simulink model "RM3_Hydraulic_PTO_HeavingSurging4"  (R2019b)
settings: Solver=ode14x  StartTime=0  StopTime=250  FixedStep=0.01  MaxStep=0.01  RelTol=1e-3  EnableMultiTasking=on
values from neighbouring files (symbols this model uses):
  simu = simulationClass()    [wecSimInputFile.m]
  waves = waveClass('regular')    [wecSimInputFile.m]
undefined symbols (not defined in the file or in its folder): body, constraint, pto, X, Y, Z
libraries: nesl_utility x73, sm_lib x40, WECSim_Lib x8, vrlib x1
(part 4 of 4)

== matlab function RM3_Hydraulic_PTO_HeavingSurging4/buoy/Hydrodynamic Body/Nonlinear Wave Elevation/Linear or Instantaneous Free Surface/Instantaneous Water Free Surface  /Instantaneous FS ==
  data: x input; center input; f output; cg input; AH input; w input; dw input; k input; typeNum input; t input; rampT input; phaseRand input; waveDir input
function f  = waveElevation(x,center,cg,AH,w,dw,k,typeNum,t,rampT,phaseRand,waveDir)
% Function to calculate the wave elevation at the ceontroids of triangulated surface
% NOTE: This function assumes that the STL file is imported with its CG at 0,0,0
f = calc_elev(x,center,cg,AH,w,dw,k,typeNum,t,rampT,phaseRand, waveDir);
end

function f = calc_elev(x,center,cg,AH,w,dw,k,typeNum,t,rampT,phaseRand,waveDir)
% Function to rotate and translate body and call wave elevation function at new locations

% Compute new tri center coords after cog rotation and translation
center = rotateXYZ(center,[1 0 0],x(4));
center = rotateXYZ(center,[0 1 0],x(5));
center = rotateXYZ(center,[0 0 1],x(6));
center = offsetXYZ(center,x);
center = offsetXYZ(center,cg);
% Calculate the free surface
f=waveElev(center,AH,w,dw,t,k,rampT,phaseRand,typeNum,waveDir);
end

function verts = offsetXYZ(verts,x)
% Function to move the position vertices
verts(:,1) = verts(:,1) + x(1);
verts(:,2) = verts(:,2) + x(2);
verts(:,3) = verts(:,3) + x(3);
end

function xn = rotateXYZ(x,ax,t)
% Function to rotate a point about an arbitrary axis
% x: 3-component coordinates
% ax: axis about which to rotate (must be a vector length 1)
% t: rotation angle
% xn: new coordinates after rotation
rotMat = zeros(3);
rotMat(1,1) = ax(1)*ax(1)*(1-cos(t))    + cos(t);
rotMat(1,2) = ax(2)*ax(1)*(1-cos(t))    + ax(3)*sin(t);
rotMat(1,3) = ax(3)*ax(1)*(1-cos(t))    - ax(2)*sin(t);
rotMat(2,1) = ax(1)*ax(2)*(1-cos(t))    - ax(3)*sin(t);
rotMat(2,2) = ax(2)*ax(2)*(1-cos(t))    + cos(t);
rotMat(2,3) = ax(3)*ax(2)*(1-cos(t))    + ax(1)*sin(t);
rotMat(3,1) = ax(1)*ax(3)*(1-cos(t))    + ax(2)*sin(t);
rotMat(3,2) = ax(2)*ax(3)*(1-cos(t))    - ax(1)*sin(t);
rotMat(3,3) = ax(3)*ax(3)*(1-cos(t))    + cos(t);
xn = x*rotMat;
end

function f=waveElev(center,AH,w,dw,t,k,rampT,phaseRand,typeNum,waveDir)
% Function to calculate the wave elevation at an array of points
f = zeros(length(center(:,3)),1);
cx = center(:,1);
cy = center(:,2);
X = cx*cos(waveDir*pi/180) + cy*sin(waveDir*pi/180);
if typeNum <10
elseif typeNum <20
    f = AH(1).*cos(k(1).*X-w(1)*t);
elseif typeNum <30
    tmp=sqrt(AH.*dw);
    tmp1 = ones(1,length(center(:,1)));
    tmp2 = (w.*t+phaseRand)*tmp1;
    tmp3 = cos(k*X'- tmp2);
    f(:,1) = tmp3'*tmp;
end
if t<=rampT
    rampF = (1+cos(pi+pi*t/rampT))/2;
    f = f.*rampF;
end
end

== matlab function RM3_Hydraulic_PTO_HeavingSurging4/buoy/Hydrodynamic Body/Structure/Motion Sensor/Angle ==
  data: Q input; E output
function E  = quaternion2eulerxyz(Q)
% Takes the orientation of the body in quaternion format and converts it to
% Euler/Tait-Bryan/Cardan angles in the XYZ convention: roll [-180,180],
% followed by pitch [-90,90], followed by yaw [-180,180].
E = zeros(3,1);

E(1) = atan2(-2 * ( Q(3)*Q(4) - Q(1)*Q(2)), (Q(1)^2 - Q(2)^2 - Q(3)^2 + Q(4)^2));
E(2) = asin(2 *   ( Q(2)*Q(4) + Q(1)*Q(3)));
E(3) = atan2(-2 * ( Q(2)*Q(3) - Q(1)*Q(4)), (Q(1)^2 + Q(2)^2 - Q(3)^2 - Q(4)^2));

% E(1) = atan2((2*(Q(1)*Q(2)+Q(3)*Q(4))),(1-2*(Q(2)^2+Q(3)^2)));
% E(2) = asin(2*(Q(1)*Q(3)-Q(4)*Q(2)));
% E(3) = atan2((2*(Q(1)*Q(4)+Q(2)*Q(3))),(1-2*(Q(3)^2+Q(4)^2)));

== matlab function RM3_Hydraulic_PTO_HeavingSurging4/buoy/Hydrodynamic Body/Wave Diffraction and Excitation Force Calculation/Linear Wave Excitation Force Variant Subsystem/Irregular Wave Excitation Force/MATLAB Function ==
  data: A input; Fext output; w input; fExtRE input; fExtIM input; phaseRand input; dw input; time input; WaveDir input; WaveSpread input; fExtMD input
function Fext = fcn(A,w,fExtRE,fExtIM,phaseRand,dw,time,WaveDir,WaveSpread,fExtMD)
%#codegen

% pversistent A1 B1 B11 C1 D1 D11 E1 E11

A1=bsxfun(@plus,w*time,pi/2);
Fext = zeros(1,6);
for ii=1:length(WaveDir)
    B1= sin(bsxfun(@plus,A1,phaseRand(:,ii)));
    B11 = sin(bsxfun(@plus,w*time,phaseRand(:,ii)));
    C0 = bsxfun(@times,A*WaveSpread(ii),dw);
    C1 = sqrt(bsxfun(@times,A*WaveSpread(ii),dw));
    D0 =bsxfun(@times,squeeze(fExtMD(ii,:,:)),C0);
    D1 =bsxfun(@times,squeeze(fExtRE(ii,:,:)),C1);
    D11 = bsxfun(@times,squeeze(fExtIM(ii,:,:)),C1);
    E1 = D0+ bsxfun(@times,B1,D1);
    E11 = bsxfun(@times,B11,D11);
    Fext = Fext + sum(bsxfun(@minus,E1,E11));
end

== matlab function RM3_Hydraulic_PTO_HeavingSurging4/buoy/Hydrodynamic Body/Wave Diffraction and Excitation Force Calculation/Nonlinear FK Force Variant Subsystem/With Nonlinear FroudeKrylov Force/Diffraction and Excitation Forces ==
  data: x input; elv input; center input; f output; tnorm input; area input; rho input; g input; cg input; AH input; w input; dw input; wDepth input; deepWaterWave input; k input; typeNum input; t input; phaseRand input; wp output; wpMeanFS output
function [f, wp, wpMeanFS]  = nonFKForce(x,elv,center,tnorm,area,rho,g,cg,AH,w,dw,wDepth,deepWaterWave,k,typeNum,t,phaseRand)
% Function to calculate wave exitation force and moment on a triangulated surface
% NOTE: This function assumes that the STL file is imported with its CG at 0,0,0

% Logic to calculate nonFKForce at reduced sample time
[f, wp, wpMeanFS] = calc_force(x,elv,center,tnorm,area,rho,g,cg,AH,w,dw,wDepth,deepWaterWave,k,typeNum,t,phaseRand);
end

function [f, wp, wpMeanFS]  = calc_force(x,elv,center,tnorm,area,rho,g,cg,AH,w,dw,wDepth,deepWaterWave,k,typeNum,t,phaseRand)
% Function to apply translation and rotation, and calculate forces.

% Compute new tri coords after cog rotation and translation
centerMeanFS = offsetXYZ(center,cg);
avMeanFS     = tnorm .* [area area area];

% Compute new tri coords after cog rotation and translation
center = rotateXYZ(center,[1 0 0],x(4));
center = rotateXYZ(center,[0 1 0],x(5));
center = rotateXYZ(center,[0 0 1],x(6));
center = offsetXYZ(center,x);
center = offsetXYZ(center,cg);
% Compute new normal vectors coords after cog rotation and translation
tnorm = rotateXYZ(tnorm,[1 0 0],x(4));
tnorm = rotateXYZ(tnorm,[0 1 0],x(5));
tnorm = rotateXYZ(tnorm,[0 0 1],x(6));

% Copute area vectors
av = tnorm .* [area area area];

% Calculate the free surface
wpMeanFS=pDis(centerMeanFS,       0,AH,w,dw,wDepth,deepWaterWave,t,k,phaseRand,typeNum,rho,g);
wp      =pDis(center      ,     elv,AH,w,dw,wDepth,deepWaterWave,t,k,phaseRand,typeNum,rho,g);

% Calculate forces
f_linear   =FK(centerMeanFS,       cg,avMeanFS,wpMeanFS);
f_nonLinear=FK(center      ,x(1:3)+cg,av      ,wp      );
f = f_nonLinear-f_linear;
end

function verts = offsetXYZ(verts,x)
% Function to move the position vertices
verts(:,1) = verts(:,1) + x(1);
verts(:,2) = verts(:,2) + x(2);
verts(:,3) = verts(:,3) + x(3);
end

function xn = rotateXYZ(x,ax,t)
% Function to rotate a point about an arbitrary axis
% x: 3-componenet coordinates
% ax: axis about which to rotate (must be a vector length 1)
% t: rotation angle
% xn: new coordinates after rotation
rotMat = zeros(3);
rotMat(1,1) = ax(1)*ax(1)*(1-cos(t))    + cos(t);
rotMat(1,2) = ax(2)*ax(1)*(1-cos(t))    + ax(3)*sin(t);
rotMat(1,3) = ax(3)*ax(1)*(1-cos(t))    - ax(2)*sin(t);
rotMat(2,1) = ax(1)*ax(2)*(1-cos(t))    - ax(3)*sin(t);
rotMat(2,2) = ax(2)*ax(2)*(1-cos(t))    + cos(t);
rotMat(2,3) = ax(3)*ax(2)*(1-cos(t))    + ax(1)*sin(t);
rotMat(3,1) = ax(1)*ax(3)*(1-cos(t))    + ax(2)*sin(t);
rotMat(3,2) = ax(2)*ax(3)*(1-cos(t))    - ax(1)*sin(t);
rotMat(3,3) = ax(3)*ax(3)*(1-cos(t))    + cos(t);
xn = x*rotMat;
end

function f=pDis(center,elv,AH,w,dw,wDepth,deepWaterWave,t,k,phaseRand,typeNum,rho,g)
% Function to calculate pressure distribution
f = zeros(length(center(:,3)),1);
z=zeros(length(center(:,1)),1);
if typeNum <10
elseif typeNum <20
    f = rho.*g.*AH(1).*cos(k(1).*center(:,1)-w(1)*t);
    if deepWaterWave == 0
        z=(center(:,3)-elv).*wDepth./(wDepth+elv);
        f = f.*(cosh(k(1).*(z+wDepth))./cosh(k(1)*wDepth));
    else
        z=(center(:,3)-elv);
        f = f.*exp(k(1).*z);
    end
elseif typeNum <30
    for i=1:length(AH)
        if deepWaterWave == 0 && wDepth <= 0.5*pi/k(i)
            z=(center(:,3)-elv).*wDepth./(wDepth+elv);
            f_tmp = rho.*g.*sqrt(AH(i)*dw(i)).*cos(k(i).*center(:,1)-w(i)*t-phaseRand(i));
            f = f + f_tmp.*(cosh(k(i).*(z+wDepth))./cosh(k(i).*wDepth));
        else
            z=(center(:,3)-elv);
            f_tmp = rho.*g.*sqrt(AH(i)*dw(i)).*cos(k(i).*center(:,1)-w(i)*t-phaseRand(i));
            f = f + f_tmp.*exp(k(i).*z);
        end
    end
end
f(z>0)=0;
end

function f = FK(center,instcg,av,wp)
% Function to calculate the force and moment about the cog due to Froude-Krylov pressure
f = zeros(6,1);

% Calculate the hydrostatic pressure at each triangle center
pressureVect = [wp wp wp].*-av;

% Compute force about cog
f(1:3) = sum(pressureVect);

% Compute moment about cog
tmp1 = ones(length(center(:,1)),1);
tmp2 = tmp1*instcg';
center2cgVec = center-tmp2;

f(4:6)= sum(cross(center2cgVec,pressureVect));
end

== matlab function RM3_Hydraulic_PTO_HeavingSurging4/buoy/Hydrodynamic Body/Wave Radiation Forces Calculation/SS CI and Constant-Damping-CoeVariant Subsystem/Convolution Integral Calculation/MATLAB Function1 ==
  data: v input; F_FM output; IRKB input; lenJ input; CTTime input
function F_FM = ConvolutionIntegral_interp(v, IRKB, lenJ, CTTime)
%#codegen
% Function to calculate convolution integral

%define persistent variables
interp_factor = 1;
persistent velocity IRKB_interp CTTime_interp;

if isempty(velocity) 
    CTTime_interp  = CTTime(1:interp_factor:end);
    velocity       = zeros(lenJ,length(CTTime_interp));
    IRKB_reordered = permute(IRKB,[3 1 2]);                     % permutes from [601 6 12] to [12 601 6]
    IRKB_interp    = IRKB_reordered(:,1:interp_factor:end, :);  % what does this do?
end 
% shift velocity
velocity      = circshift(velocity, 1, 2);
v = v(:)'';           %force v to be a column
velocity(:,1) = v(:);

%integrate
time_series = bsxfun(@times, IRKB_interp, velocity);
F_FM = squeeze(trapz(CTTime_interp,sum(time_series, 1)));

end

== matlab function RM3_Hydraulic_PTO_HeavingSurging4/buoy/Non-Hydro Body/Structure/Motion Sensor/Angle ==
  data: Q input; E output
function E  = EulerAngle(Q)
% Euler Angle Type II or Tait-Bryan Angle for sequence 321 or zyx (Nautical or Cardan angles).
% Yaw [-180,180], followed by pitch [-90,90], followed by roll [-180,180]
E = zeros(3,1);
E(1) = atan2( (2*(Q(1)*Q(2)+Q(3)*Q(4))), (1-2* (Q(2)^2+Q(3)^2) ) );
E(2) = asin( 2* (Q(1)*Q(3) - Q(4)*Q(2)));
E(3) = atan2( (2*(Q(1)*Q(4)+Q(2)*Q(3))), (1-2* (Q(3)^2+Q(4)^2) ) );
